simulink model "shorttransmissionlnewithtags"  (R2024b)
settings: Solver=VariableStepAuto  StartTime=0.0  StopTime=1  RelTol=1e-3
libraries: spsRMSLib x8, spsPower3phInstantaneousLib x2, spsThreePhaseVIMeasurementLib x2, spsThreePhaseSourceLib x1, spsThreePhaseParallelRLCLoadLib x1, spsThreePhaseSeriesRLCBranchLib x1, sps_lib x1
settings Model: Creator=brain  LastModifiedBy=brain

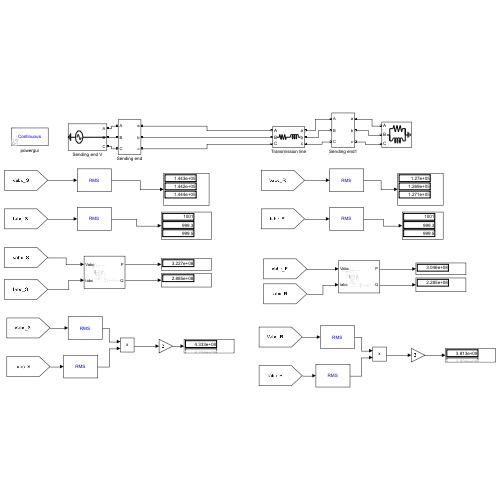
[thumbnail: Simulink's stored preview of the top-level diagram]
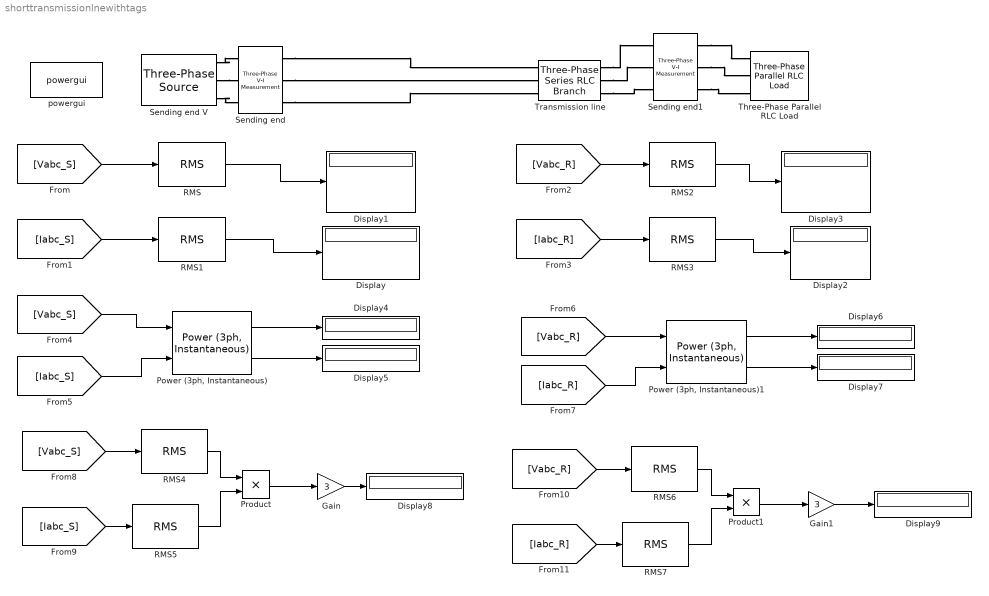
== system shorttransmissionlnewithtags ==
  Display{,1..9} (10 alike) : Display
  Gain : Gain  Gain=3
  Gain1 : Gain  Gain=3
  "Power (3ph, Instantaneous)" : spsPower3phInstantaneousLib/Power (3ph, Instantaneous)
  "Power (3ph, Instantaneous)1" : spsPower3phInstantaneousLib/Power (3ph, Instantaneous)
  Product : Product
  Product1 : Product
  RMS{,1..7} (8 alike) : spsRMSLib/RMS  TrueRMS=on  Freq=60  RMSInit=0  Ts=0
  Sending end : spsThreePhaseVIMeasurementLib/Three-Phase V-I Measurement  VoltageMeasurement=phase-to-ground  SetLabelV=on  LabelV=Vabc_S  Vpu=off  VpuLL=off  CurrentMeasurement=yes  SetLabelI=on  LabelI=Iabc_S  Ipu=off  Pbase=100e6  Vbase=500e3  OutputType=Complex  PhasorSimulation=off  PSBequivalent=0
  Sending end V : spsThreePhaseSourceLib/Three-Phase Source  InternalConnection=Yg  VoltagePhases=off  Voltage=250e3  PhaseAngle=0  Voltage_phases=[25e3 25e3 25e3]/sqrt(3)  PhaseAngles_phases=[0 -120 +120]  Frequency=60  NonIdealSource=on  SpecifyImpedance=off  Resistance=0  Inductance=0  ShortCircuitLevel=100e6  BaseVoltage=250e3  XRratio=7  BusType=swing  Pref=10e3  Qref=0  Prefabc=[10e3, 10e3, 10e3]  Qrefabc=[0, 0, 0]  Qmin=-inf  Qmax=inf
  Sending end1 : spsThreePhaseVIMeasurementLib/Three-Phase V-I Measurement  VoltageMeasurement=phase-to-ground  SetLabelV=on  LabelV=Vabc_R  Vpu=off  VpuLL=off  CurrentMeasurement=yes  SetLabelI=on  LabelI=Iabc_R  Ipu=off  Pbase=100e6  Vbase=500e3  OutputType=Complex  PhasorSimulation=off  PSBequivalent=0
  Three-Phase Parallel RLC Load : spsThreePhaseParallelRLCLoadLib/Three-Phase Parallel RLC Load  LConnTagsString=A|B|C  Configuration=Y (grounded)  NominalVoltage=220e3  Vabc=[1e3 1e3 1e3]  Vabcp=[1e3 1e3 1e3]  NominalFrequency=60  UnbalancedPower=off  ActivePower=304.8e6  InductivePower=228.6e6  CapacitivePower=0  Pabc=[10e3 9e3 11e3]  QLabc=[100 90 110]  QCabc=[100 90 110]  Pabcp=[10e3 9e3 11e3]  QLabcp=[100 90 110]  QCabcp=[100 90 110]  Measurements=None  LoadType=constant Z
  Transmission line : spsThreePhaseSeriesRLCBranchLib/Three-Phase Series RLC Branch  LConnTagsString=A|B|C  RConnTagsString=A|B|C  BranchType=RL  Resistance=6  Inductance=0.053052  Capacitance=1e-6  Measurements=None
  powergui : sps_lib/powergui  Priority=1  SimulationMode=Continuous  SampleTime=50e-6  frequency=60  Iterations=50  frequencyindice=60  Pbase=100e6  ErrMax=1e-4  UnitsV=kV  UnitsW=MW  buscounter=0  FunctionMessages=off  echomessages=off  EnableUseOfTLC=off  CurrentSourceSwitches=off  DisableSnubberDevices=off  DisableRonSwitches=off  DisableVfSwitches=off  DisplayEquations=off  AutomaticDiscreteSolvers=off  SolverType=Tustin/Backward Euler (TBE)  Interpol=off  ExternalGateDelay=off  methode=off  Ts=100  x0status=blocks  SPID=on  SwTol=0  HookPort=off  NonlinearTolerance=1e-4  nMaxIteration=100  ContinueOnMaxIteration=off  RestoreLinks=warning  ResistiveCurrentMeasurement=off  Frange=[0:2:500]  Ylog=off  Xlog=on  ShowGrid=off  save=off  variable=ZData  structure=0  ZoomFFT=off  StartTime=0.0  cycles=1  DisplayStyle=1  fundamental=60  FreqAxis=off  MaxFrequency=1000  frequencyindicesteady=1  RmsSteady=1  display=off
  wires:
  [Vabc_S] -> RMS/1
  RMS/1 -> Display1/1
  [Iabc_S] -> RMS1/1
  RMS1/1 -> Display/1
  RMS3/1 -> Display2/1
  [Iabc_R] -> RMS3/1
  RMS2/1 -> Display3/1
  [Vabc_R] -> RMS2/1
  [Vabc_S] -> "Power (3ph, Instantaneous)"/1
  [Iabc_S] -> "Power (3ph, Instantaneous)"/2
  "Power (3ph, Instantaneous)"/1 -> Display4/1
  "Power (3ph, Instantaneous)"/2 -> Display5/1
  "Power (3ph, Instantaneous)1"/2 -> Display7/1
  "Power (3ph, Instantaneous)1"/1 -> Display6/1
  [Iabc_R] -> "Power (3ph, Instantaneous)1"/2
  [Vabc_R] -> "Power (3ph, Instantaneous)1"/1
  [Iabc_S] -> RMS5/1
  [Vabc_S] -> RMS4/1
  RMS4/1 -> Product/1
  RMS5/1 -> Product/2
  Product/1 -> Gain/1
  Gain/1 -> Display8/1
  Gain1/1 -> Display9/1
  Product1/1 -> Gain1/1
  RMS7/1 -> Product1/2
  RMS6/1 -> Product1/1
  [Vabc_R] -> RMS6/1
  [Iabc_R] -> RMS7/1
  connections:
  Sending end V/RConn1 -- Sending end/LConn1
  Sending end V/RConn2 -- Sending end/LConn2
  Sending end V/RConn3 -- Sending end/LConn3
  Sending end/RConn1 -- Transmission line/LConn1
  Sending end/RConn2 -- Transmission line/LConn2
  Sending end/RConn3 -- Transmission line/LConn3
  Transmission line/RConn1 -- Sending end1/LConn1
  Transmission line/RConn3 -- Sending end1/LConn3
  Transmission line/RConn2 -- Sending end1/LConn2
  Sending end1/RConn1 -- Three-Phase Parallel RLC Load/LConn1
  Sending end1/RConn2 -- Three-Phase Parallel RLC Load/LConn2
  Sending end1/RConn3 -- Three-Phase Parallel RLC Load/LConn3
